simulink model "exampleModel_bus_axi_w_4ptavg"  (R2017b)
settings: Solver=VariableStepAuto  StartTime=0.0  StopTime=10e-5  RelTol=1e-3
PreLoadFcn:
  | setup
values from neighbouring files (symbols this model uses):
  axiClk = 156.25e6    (= 156250000)    [setup.m]    (also in setup_exampleModel_bus_axi_simulink.m; setup_exampleModel_bus_axi_simulink_lcls2.m; setup_lcls2_pcav.m; sysgen_signal.m)
  cav1p1_addr = 204    [setup_exampleModel_bus_axi_simulink.m]    (also in setup_exampleModel_bus_axi_simulink_lcls2.m; setup_lcls2_pcav.m; sysgen_signal.m)
  cav1p2_addr = cav1p1_addr * 2    (= 408)    [setup_exampleModel_bus_axi_simulink.m]    (also in setup_exampleModel_bus_axi_simulink_lcls2.m; setup_lcls2_pcav.m; sysgen_signal.m)
  cav2p1_addr = cav1p1_addr * 3    (= 612)    [setup_exampleModel_bus_axi_simulink.m]    (also in setup_exampleModel_bus_axi_simulink_lcls2.m; setup_lcls2_pcav.m; sysgen_signal.m)
  cav2p2_addr = cav1p1_addr * 4    (= 816)    [setup_exampleModel_bus_axi_simulink.m]    (also in setup_exampleModel_bus_axi_simulink_lcls2.m; setup_lcls2_pcav.m; sysgen_signal.m)
  Fadc = Fs/interleavedChannels    (= 29750000)    [setup.m]    (also in setup_exampleModel_bus_axi_simulink.m = 357000000; setup_exampleModel_bus_axi_simulink_lcls2.m = 351000000; setup_lcls2_pcav.m = 357000000; sysgen_signal.m = 357000000)
  fir_lpf = fir1(15, w_lpf)    [setup_exampleModel_bus_axi_simulink.m]    (also in setup_exampleModel_bus_axi_simulink_lcls2.m; setup_lcls2_pcav.m)
  Fproc = 204e6    (= 204000000)    [setup_exampleModel_bus_axi_simulink.m]    (also in setup_exampleModel_bus_axi_simulink_lcls2.m = 200571400; setup_lcls2_pcav.m; sysgen_signal.m)
  Fsig = Fproc/12    (= 17000000)    [setup_exampleModel_bus_axi_simulink.m]    (also in setup_exampleModel_bus_axi_simulink_lcls2.m = 16714283.3333; setup_lcls2_pcav.m)
  Tadc = 1/fadc    (= 2.80112044818e-09)    [cavity_signal.m]    (also in setup_exampleModel_bus_axi_simulink.m; setup_exampleModel_bus_axi_simulink_lcls2.m = 2.849002849e-09; setup_lcls2_pcav.m; setup_pcav_simulink.m)
undefined symbols (not defined in the file or in its folder): AXI4, Lite
libraries: xbsIndex_r4 x2870, llrf_lib x10, simulink x3
(part 4 of 15)

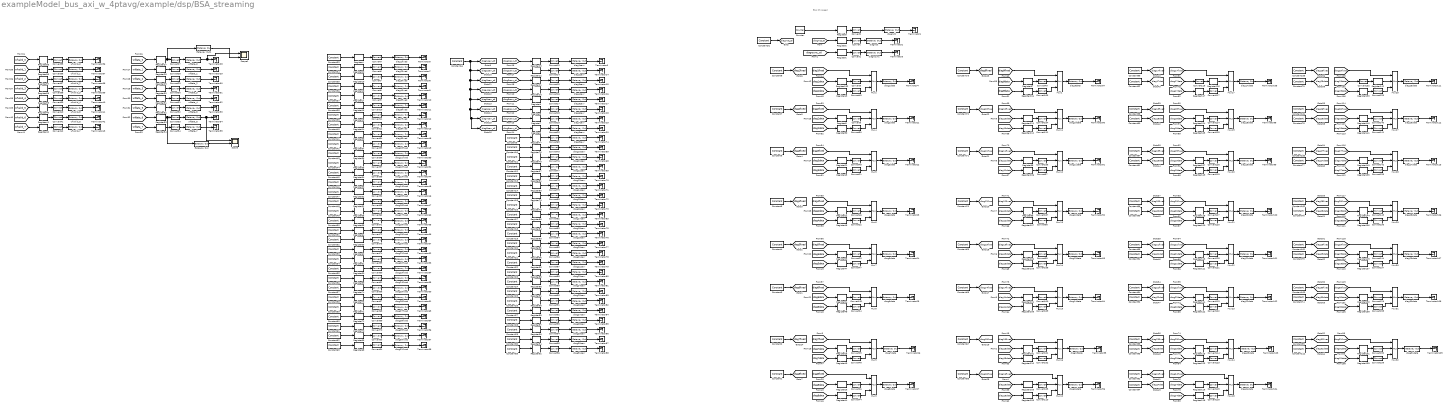
== system exampleModel_bus_axi_w_4ptavg/example/dsp/BSA_streaming ==
  note: BSA Clk speed
  Constant{1..8,66..73,82..89,99..105} (31 alike) : xbsIndex_r4/Constant  const=0  gui_display_data_type=Boolean  arith_type=Boolean  n_bits=16  bin_pt=14  preci_type=Single  exp_width=8  frac_width=24  explicit_period=off  period=1  equ=P=C  opselect=C  inp2=PCIN>>17  opr=+  inp1=P  carry=CIN  dbl_ovrd=off  block_type=constant
  Constant{9..30,64..65} (24 alike) : xbsIndex_r4/Constant  const=0  gui_display_data_type=Fixed-point  arith_type=Unsigned  n_bits=3  bin_pt=0  preci_type=Single  exp_width=8  frac_width=24  explicit_period=on  period=1/(17e6)  equ=P=C  opselect=C  inp2=PCIN>>17  opr=+  inp1=P  carry=CIN  dbl_ovrd=off  block_type=constant
  Constant{32,74..81,90..94,112} (15 alike) : xbsIndex_r4/Constant  const=0  gui_display_data_type=Fixed-point  arith_type=Signed (2's comp)  n_bits=18  bin_pt=0  preci_type=Single  exp_width=8  frac_width=24  explicit_period=on  period=1/Fproc  equ=P=C  opselect=C  inp2=PCIN>>17  opr=+  inp1=P  carry=CIN  dbl_ovrd=off  block_type=constant
  Constant31 : xbsIndex_r4/Constant  const=0  gui_display_data_type=Boolean  arith_type=Boolean  n_bits=16  bin_pt=14  preci_type=Single  exp_width=8  frac_width=24  explicit_period=on  period=1/(17e6)  equ=P=C  opselect=C  inp2=PCIN>>17  opr=+  inp1=P  carry=CIN  dbl_ovrd=off  block_type=constant
  Constant{33..63} (31 alike) : xbsIndex_r4/Constant  const=0  gui_display_data_type=Fixed-point  arith_type=Unsigned  n_bits=1  bin_pt=0  preci_type=Single  exp_width=8  frac_width=24  explicit_period=on  period=1/(17e6)  equ=P=C  opselect=C  inp2=PCIN>>17  opr=+  inp1=P  carry=CIN  dbl_ovrd=off  block_type=constant
  Convert{,1,4,6..12,35..42,51..64,66..74} (41 alike) : xbsIndex_r4/Convert  gui_display_data_type=Boolean  arith_type=Boolean  n_bits=16  bin_pt=14  float_type=Single  exp_bits=8  fraction_bits=24  quantization=Truncate  overflow=Wrap  en=off  latency=1  pipeline=off  dbl_ovrd=off  block_type=convert
  Convert{3,25,46,49,100..101,107,131} (8 alike) : xbsIndex_r4/Convert  gui_display_data_type=Fixed-point  arith_type="Signed  (2's comp)"  n_bits=18  bin_pt=16  float_type=Single  exp_bits=8  fraction_bits=24  quantization=Truncate  overflow=Wrap  en=off  latency=1  pipeline=off  dbl_ovrd=off  block_type=convert
  Convert{22,24,29..32,34,43,48,98,102..103,109} (13 alike) : xbsIndex_r4/Convert  gui_display_data_type=Fixed-point  arith_type="Signed  (2's comp)"  n_bits=32  bin_pt=16  float_type=Single  exp_bits=8  fraction_bits=24  quantization=Truncate  overflow=Wrap  en=off  latency=1  pipeline=off  dbl_ovrd=off  block_type=convert
  Convert{5,45,104,106} (4 alike) : xbsIndex_r4/Convert  gui_display_data_type=Fixed-point  arith_type="Signed  (2's comp)"  n_bits=18  bin_pt=15  float_type=Single  exp_bits=8  fraction_bits=24  quantization=Truncate  overflow=Wrap  en=off  latency=1  pipeline=off  dbl_ovrd=off  block_type=convert
  Convert{23,26,99,105,113..116,124,126..130,132,140,142..144} (19 alike) : xbsIndex_r4/Convert  gui_display_data_type=Fixed-point  arith_type="Signed  (2's comp)"  n_bits=18  bin_pt=0  float_type=Single  exp_bits=8  fraction_bits=24  quantization=Truncate  overflow=Wrap  en=off  latency=1  pipeline=off  dbl_ovrd=off  block_type=convert
  Convert{33,44,47,108,110,117..123,125,133,135..139,141} (20 alike) : xbsIndex_r4/Convert  gui_display_data_type=Fixed-point  arith_type="Signed  (2's comp)"  n_bits=32  bin_pt=0  float_type=Single  exp_bits=8  fraction_bits=24  quantization=Truncate  overflow=Wrap  en=off  latency=1  pipeline=off  dbl_ovrd=off  block_type=convert
  Convert{21,50,97,111} (4 alike) : xbsIndex_r4/Convert  gui_display_data_type=Fixed-point  arith_type="Signed  (2's comp)"  n_bits=32  bin_pt=15  float_type=Single  exp_bits=8  fraction_bits=24  quantization=Truncate  overflow=Wrap  en=off  latency=1  pipeline=off  dbl_ovrd=off  block_type=convert
  Convert{13..20,65,75..96} (31 alike) : xbsIndex_r4/Convert  gui_display_data_type=Fixed-point  arith_type=Unsigned  n_bits=2  bin_pt=0  float_type=Single  exp_bits=8  fraction_bits=24  quantization=Truncate  overflow=Wrap  en=off  latency=1  pipeline=off  dbl_ovrd=off  block_type=convert
  Convert2 : xbsIndex_r4/Convert  gui_display_data_type=Fixed-point  arith_type=Unsigned  n_bits=1  bin_pt=0  float_type=Single  exp_bits=8  fraction_bits=24  quantization=Truncate  overflow=Saturate  en=off  latency=1  pipeline=off  dbl_ovrd=off  block_type=convert
  Convert27 : xbsIndex_r4/Convert  gui_display_data_type=Fixed-point  arith_type="Signed  (2's comp)"  n_bits=32  bin_pt=24  float_type=Single  exp_bits=8  fraction_bits=24  quantization=Truncate  overflow=Wrap  en=off  latency=1  pipeline=off  dbl_ovrd=off  block_type=convert
  Convert28 : xbsIndex_r4/Convert  gui_display_data_type=Fixed-point  arith_type="Signed  (2's comp)"  n_bits=32  bin_pt=24  float_type=Single  exp_bits=8  fraction_bits=24  quantization=Truncate  overflow=Wrap  en=off  latency=1  pipeline=off  dbl_ovrd=off  block_type=convert
  Counter : xbsIndex_r4/Counter  cnt_type=Free Running  cnt_to=Inf  operation=Up  start_count=0  cnt_by_val=1  arith_type=Unsigned  n_bits=1  bin_pt=0  load_pin=off  rst=off  en=off  explicit_period=on  period=1/(Fproc)  use_behavioral_HDL=off  implementation=Fabric  dbl_ovrd=off  block_type=counter
  Gateway Out : xbsIndex_r4/Gateway Out  inherit_from_input=off  hdl_port=on  rows=1  columns=1  UseAsDAC=off  DACChannel='1'  interface=None  automatic_assignment=on  address_offset=hex2dec('00')  intf_name=''  intf_description=''  timing_constraint=None  locs_specified=off  LOCs={}  io_standard={}  block_type=gatewayout
  Gateway Out1 : xbsIndex_r4/Gateway Out  inherit_from_input=off  hdl_port=on  rows=1  columns=1  UseAsDAC=off  DACChannel='1'  interface=None  automatic_assignment=on  address_offset=hex2dec('00')  intf_name=''  intf_description=''  timing_constraint=None  locs_specified=off  LOCs={}  io_standard={}  block_type=gatewayout
  Mux{1..25,27..32} (31 alike) : xbsIndex_r4/Mux  inputs=2  en=off  latency=1  precision=Full  arith_type=Unsigned  n_bits=16  bin_pt=14  quantization=Truncate  overflow=Wrap  dbl_ovrd=off  block_type=mux
  Register{1..133,135..144} (143 alike) : xbsIndex_r4/Register  init=0  rst=off  en=off  dbl_ovrd=off  block_type=register
  Scope : Scope  NumInputPorts=2
  Scope1 : Scope  NumInputPorts=2
  Terminator{1..109,111..113} (112 alike) : Terminator
  diag10data : xbsIndex_r4/Gateway Out  inherit_from_input=off  hdl_port=on  rows=1  columns=1  UseAsDAC=off  DACChannel='1'  interface=None  automatic_assignment=on  address_offset=hex2dec('00')  intf_name=''  intf_description=''  timing_constraint=None  locs_specified=off  LOCs={}  io_standard={}  block_type=gatewayout
  diag10fixed : xbsIndex_r4/Gateway Out  inherit_from_input=off  hdl_port=on  rows=1  columns=1  UseAsDAC=off  DACChannel='1'  interface=None  automatic_assignment=on  address_offset=hex2dec('00')  intf_name=''  intf_description=''  timing_constraint=None  locs_specified=off  LOCs={}  io_standard={}  block_type=gatewayout
  diag10sevr : xbsIndex_r4/Gateway Out  inherit_from_input=off  hdl_port=on  rows=1  columns=1  UseAsDAC=off  DACChannel='1'  interface=None  automatic_assignment=on  address_offset=hex2dec('00')  intf_name=''  intf_description=''  timing_constraint=None  locs_specified=off  LOCs={}  io_standard={}  block_type=gatewayout
  diag11data : xbsIndex_r4/Gateway Out  inherit_from_input=off  hdl_port=on  rows=1  columns=1  UseAsDAC=off  DACChannel='1'  interface=None  automatic_assignment=on  address_offset=hex2dec('00')  intf_name=''  intf_description=''  timing_constraint=None  locs_specified=off  LOCs={}  io_standard={}  block_type=gatewayout
  diag11fixed : xbsIndex_r4/Gateway Out  inherit_from_input=off  hdl_port=on  rows=1  columns=1  UseAsDAC=off  DACChannel='1'  interface=None  automatic_assignment=on  address_offset=hex2dec('00')  intf_name=''  intf_description=''  timing_constraint=None  locs_specified=off  LOCs={}  io_standard={}  block_type=gatewayout
  diag11sevr : xbsIndex_r4/Gateway Out  inherit_from_input=off  hdl_port=on  rows=1  columns=1  UseAsDAC=off  DACChannel='1'  interface=None  automatic_assignment=on  address_offset=hex2dec('00')  intf_name=''  intf_description=''  timing_constraint=None  locs_specified=off  LOCs={}  io_standard={}  block_type=gatewayout
  diag12data : xbsIndex_r4/Gateway Out  inherit_from_input=off  hdl_port=on  rows=1  columns=1  UseAsDAC=off  DACChannel='1'  interface=None  automatic_assignment=on  address_offset=hex2dec('00')  intf_name=''  intf_description=''  timing_constraint=None  locs_specified=off  LOCs={}  io_standard={}  block_type=gatewayout
  diag12fixed : xbsIndex_r4/Gateway Out  inherit_from_input=off  hdl_port=on  rows=1  columns=1  UseAsDAC=off  DACChannel='1'  interface=None  automatic_assignment=on  address_offset=hex2dec('00')  intf_name=''  intf_description=''  timing_constraint=None  locs_specified=off  LOCs={}  io_standard={}  block_type=gatewayout
  diag12sevr : xbsIndex_r4/Gateway Out  inherit_from_input=off  hdl_port=on  rows=1  columns=1  UseAsDAC=off  DACChannel='1'  interface=None  automatic_assignment=on  address_offset=hex2dec('00')  intf_name=''  intf_description=''  timing_constraint=None  locs_specified=off  LOCs={}  io_standard={}  block_type=gatewayout
  diag13data : xbsIndex_r4/Gateway Out  inherit_from_input=off  hdl_port=on  rows=1  columns=1  UseAsDAC=off  DACChannel='1'  interface=None  automatic_assignment=on  address_offset=hex2dec('00')  intf_name=''  intf_description=''  timing_constraint=None  locs_specified=off  LOCs={}  io_standard={}  block_type=gatewayout
  diag13fixed : xbsIndex_r4/Gateway Out  inherit_from_input=off  hdl_port=on  rows=1  columns=1  UseAsDAC=off  DACChannel='1'  interface=None  automatic_assignment=on  address_offset=hex2dec('00')  intf_name=''  intf_description=''  timing_constraint=None  locs_specified=off  LOCs={}  io_standard={}  block_type=gatewayout
  diag13sevr : xbsIndex_r4/Gateway Out  inherit_from_input=off  hdl_port=on  rows=1  columns=1  UseAsDAC=off  DACChannel='1'  interface=None  automatic_assignment=on  address_offset=hex2dec('00')  intf_name=''  intf_description=''  timing_constraint=None  locs_specified=off  LOCs={}  io_standard={}  block_type=gatewayout
  diag14data : xbsIndex_r4/Gateway Out  inherit_from_input=off  hdl_port=on  rows=1  columns=1  UseAsDAC=off  DACChannel='1'  interface=None  automatic_assignment=on  address_offset=hex2dec('00')  intf_name=''  intf_description=''  timing_constraint=None  locs_specified=off  LOCs={}  io_standard={}  block_type=gatewayout
  diag14fixed : xbsIndex_r4/Gateway Out  inherit_from_input=off  hdl_port=on  rows=1  columns=1  UseAsDAC=off  DACChannel='1'  interface=None  automatic_assignment=on  address_offset=hex2dec('00')  intf_name=''  intf_description=''  timing_constraint=None  locs_specified=off  LOCs={}  io_standard={}  block_type=gatewayout
  diag14sevr : xbsIndex_r4/Gateway Out  inherit_from_input=off  hdl_port=on  rows=1  columns=1  UseAsDAC=off  DACChannel='1'  interface=None  automatic_assignment=on  address_offset=hex2dec('00')  intf_name=''  intf_description=''  timing_constraint=None  locs_specified=off  LOCs={}  io_standard={}  block_type=gatewayout
  diag15data : xbsIndex_r4/Gateway Out  inherit_from_input=off  hdl_port=on  rows=1  columns=1  UseAsDAC=off  DACChannel='1'  interface=None  automatic_assignment=on  address_offset=hex2dec('00')  intf_name=''  intf_description=''  timing_constraint=None  locs_specified=off  LOCs={}  io_standard={}  block_type=gatewayout
  diag15fixed : xbsIndex_r4/Gateway Out  inherit_from_input=off  hdl_port=on  rows=1  columns=1  UseAsDAC=off  DACChannel='1'  interface=None  automatic_assignment=on  address_offset=hex2dec('00')  intf_name=''  intf_description=''  timing_constraint=None  locs_specified=off  LOCs={}  io_standard={}  block_type=gatewayout
  diag15sevr : xbsIndex_r4/Gateway Out  inherit_from_input=off  hdl_port=on  rows=1  columns=1  UseAsDAC=off  DACChannel='1'  interface=None  automatic_assignment=on  address_offset=hex2dec('00')  intf_name=''  intf_description=''  timing_constraint=None  locs_specified=off  LOCs={}  io_standard={}  block_type=gatewayout
  diag16data : xbsIndex_r4/Gateway Out  inherit_from_input=off  hdl_port=on  rows=1  columns=1  UseAsDAC=off  DACChannel='1'  interface=None  automatic_assignment=on  address_offset=hex2dec('00')  intf_name=''  intf_description=''  timing_constraint=None  locs_specified=off  LOCs={}  io_standard={}  block_type=gatewayout
  diag16fixed : xbsIndex_r4/Gateway Out  inherit_from_input=off  hdl_port=on  rows=1  columns=1  UseAsDAC=off  DACChannel='1'  interface=None  automatic_assignment=on  address_offset=hex2dec('00')  intf_name=''  intf_description=''  timing_constraint=None  locs_specified=off  LOCs={}  io_standard={}  block_type=gatewayout
  diag16sevr : xbsIndex_r4/Gateway Out  inherit_from_input=off  hdl_port=on  rows=1  columns=1  UseAsDAC=off  DACChannel='1'  interface=None  automatic_assignment=on  address_offset=hex2dec('00')  intf_name=''  intf_description=''  timing_constraint=None  locs_specified=off  LOCs={}  io_standard={}  block_type=gatewayout
  diag17data : xbsIndex_r4/Gateway Out  inherit_from_input=off  hdl_port=on  rows=1  columns=1  UseAsDAC=off  DACChannel='1'  interface=None  automatic_assignment=on  address_offset=hex2dec('00')  intf_name=''  intf_description=''  timing_constraint=None  locs_specified=off  LOCs={}  io_standard={}  block_type=gatewayout
  diag17fixed : xbsIndex_r4/Gateway Out  inherit_from_input=off  hdl_port=on  rows=1  columns=1  UseAsDAC=off  DACChannel='1'  interface=None  automatic_assignment=on  address_offset=hex2dec('00')  intf_name=''  intf_description=''  timing_constraint=None  locs_specified=off  LOCs={}  io_standard={}  block_type=gatewayout
  diag17sevr : xbsIndex_r4/Gateway Out  inherit_from_input=off  hdl_port=on  rows=1  columns=1  UseAsDAC=off  DACChannel='1'  interface=None  automatic_assignment=on  address_offset=hex2dec('00')  intf_name=''  intf_description=''  timing_constraint=None  locs_specified=off  LOCs={}  io_standard={}  block_type=gatewayout
  diag18data : xbsIndex_r4/Gateway Out  inherit_from_input=off  hdl_port=on  rows=1  columns=1  UseAsDAC=off  DACChannel='1'  interface=None  automatic_assignment=on  address_offset=hex2dec('00')  intf_name=''  intf_description=''  timing_constraint=None  locs_specified=off  LOCs={}  io_standard={}  block_type=gatewayout
  diag18fixed : xbsIndex_r4/Gateway Out  inherit_from_input=off  hdl_port=on  rows=1  columns=1  UseAsDAC=off  DACChannel='1'  interface=None  automatic_assignment=on  address_offset=hex2dec('00')  intf_name=''  intf_description=''  timing_constraint=None  locs_specified=off  LOCs={}  io_standard={}  block_type=gatewayout
  diag18sevr : xbsIndex_r4/Gateway Out  inherit_from_input=off  hdl_port=on  rows=1  columns=1  UseAsDAC=off  DACChannel='1'  interface=None  automatic_assignment=on  address_offset=hex2dec('00')  intf_name=''  intf_description=''  timing_constraint=None  locs_specified=off  LOCs={}  io_standard={}  block_type=gatewayout
  diag19data : xbsIndex_r4/Gateway Out  inherit_from_input=off  hdl_port=on  rows=1  columns=1  UseAsDAC=off  DACChannel='1'  interface=None  automatic_assignment=on  address_offset=hex2dec('00')  intf_name=''  intf_description=''  timing_constraint=None  locs_specified=off  LOCs={}  io_standard={}  block_type=gatewayout
  diag19fixed : xbsIndex_r4/Gateway Out  inherit_from_input=off  hdl_port=on  rows=1  columns=1  UseAsDAC=off  DACChannel='1'  interface=None  automatic_assignment=on  address_offset=hex2dec('00')  intf_name=''  intf_description=''  timing_constraint=None  locs_specified=off  LOCs={}  io_standard={}  block_type=gatewayout
  diag19sevr : xbsIndex_r4/Gateway Out  inherit_from_input=off  hdl_port=on  rows=1  columns=1  UseAsDAC=off  DACChannel='1'  interface=None  automatic_assignment=on  address_offset=hex2dec('00')  intf_name=''  intf_description=''  timing_constraint=None  locs_specified=off  LOCs={}  io_standard={}  block_type=gatewayout
  diag1data : xbsIndex_r4/Gateway Out  inherit_from_input=off  hdl_port=on  rows=1  columns=1  UseAsDAC=off  DACChannel='1'  interface=None  automatic_assignment=on  address_offset=hex2dec('00')  intf_name=''  intf_description=''  timing_constraint=None  locs_specified=off  LOCs={}  io_standard={}  block_type=gatewayout
  diag1fixed : xbsIndex_r4/Gateway Out  inherit_from_input=off  hdl_port=on  rows=1  columns=1  UseAsDAC=off  DACChannel='1'  interface=None  automatic_assignment=on  address_offset=hex2dec('00')  intf_name=''  intf_description=''  timing_constraint=None  locs_specified=off  LOCs={}  io_standard={}  block_type=gatewayout
  diag1sevr : xbsIndex_r4/Gateway Out  inherit_from_input=off  hdl_port=on  rows=1  columns=1  UseAsDAC=off  DACChannel='1'  interface=None  automatic_assignment=on  address_offset=hex2dec('00')  intf_name=''  intf_description=''  timing_constraint=None  locs_specified=off  LOCs={}  io_standard={}  block_type=gatewayout
  diag20data : xbsIndex_r4/Gateway Out  inherit_from_input=off  hdl_port=on  rows=1  columns=1  UseAsDAC=off  DACChannel='1'  interface=None  automatic_assignment=on  address_offset=hex2dec('00')  intf_name=''  intf_description=''  timing_constraint=None  locs_specified=off  LOCs={}  io_standard={}  block_type=gatewayout
  diag20fixed : xbsIndex_r4/Gateway Out  inherit_from_input=off  hdl_port=on  rows=1  columns=1  UseAsDAC=off  DACChannel='1'  interface=None  automatic_assignment=on  address_offset=hex2dec('00')  intf_name=''  intf_description=''  timing_constraint=None  locs_specified=off  LOCs={}  io_standard={}  block_type=gatewayout
  diag20sevr : xbsIndex_r4/Gateway Out  inherit_from_input=off  hdl_port=on  rows=1  columns=1  UseAsDAC=off  DACChannel='1'  interface=None  automatic_assignment=on  address_offset=hex2dec('00')  intf_name=''  intf_description=''  timing_constraint=None  locs_specified=off  LOCs={}  io_standard={}  block_type=gatewayout
  diag21data : xbsIndex_r4/Gateway Out  inherit_from_input=off  hdl_port=on  rows=1  columns=1  UseAsDAC=off  DACChannel='1'  interface=None  automatic_assignment=on  address_offset=hex2dec('00')  intf_name=''  intf_description=''  timing_constraint=None  locs_specified=off  LOCs={}  io_standard={}  block_type=gatewayout
  diag21fixed : xbsIndex_r4/Gateway Out  inherit_from_input=off  hdl_port=on  rows=1  columns=1  UseAsDAC=off  DACChannel='1'  interface=None  automatic_assignment=on  address_offset=hex2dec('00')  intf_name=''  intf_description=''  timing_constraint=None  locs_specified=off  LOCs={}  io_standard={}  block_type=gatewayout
  diag21sevr : xbsIndex_r4/Gateway Out  inherit_from_input=off  hdl_port=on  rows=1  columns=1  UseAsDAC=off  DACChannel='1'  interface=None  automatic_assignment=on  address_offset=hex2dec('00')  intf_name=''  intf_description=''  timing_constraint=None  locs_specified=off  LOCs={}  io_standard={}  block_type=gatewayout
  diag22data : xbsIndex_r4/Gateway Out  inherit_from_input=off  hdl_port=on  rows=1  columns=1  UseAsDAC=off  DACChannel='1'  interface=None  automatic_assignment=on  address_offset=hex2dec('00')  intf_name=''  intf_description=''  timing_constraint=None  locs_specified=off  LOCs={}  io_standard={}  block_type=gatewayout
  diag22fixed : xbsIndex_r4/Gateway Out  inherit_from_input=off  hdl_port=on  rows=1  columns=1  UseAsDAC=off  DACChannel='1'  interface=None  automatic_assignment=on  address_offset=hex2dec('00')  intf_name=''  intf_description=''  timing_constraint=None  locs_specified=off  LOCs={}  io_standard={}  block_type=gatewayout
  diag22sevr : xbsIndex_r4/Gateway Out  inherit_from_input=off  hdl_port=on  rows=1  columns=1  UseAsDAC=off  DACChannel='1'  interface=None  automatic_assignment=on  address_offset=hex2dec('00')  intf_name=''  intf_description=''  timing_constraint=None  locs_specified=off  LOCs={}  io_standard={}  block_type=gatewayout
  diag23data : xbsIndex_r4/Gateway Out  inherit_from_input=off  hdl_port=on  rows=1  columns=1  UseAsDAC=off  DACChannel='1'  interface=None  automatic_assignment=on  address_offset=hex2dec('00')  intf_name=''  intf_description=''  timing_constraint=None  locs_specified=off  LOCs={}  io_standard={}  block_type=gatewayout
  diag23fixed : xbsIndex_r4/Gateway Out  inherit_from_input=off  hdl_port=on  rows=1  columns=1  UseAsDAC=off  DACChannel='1'  interface=None  automatic_assignment=on  address_offset=hex2dec('00')  intf_name=''  intf_description=''  timing_constraint=None  locs_specified=off  LOCs={}  io_standard={}  block_type=gatewayout
  diag23sevr : xbsIndex_r4/Gateway Out  inherit_from_input=off  hdl_port=on  rows=1  columns=1  UseAsDAC=off  DACChannel='1'  interface=None  automatic_assignment=on  address_offset=hex2dec('00')  intf_name=''  intf_description=''  timing_constraint=None  locs_specified=off  LOCs={}  io_standard={}  block_type=gatewayout
  diag24data : xbsIndex_r4/Gateway Out  inherit_from_input=off  hdl_port=on  rows=1  columns=1  UseAsDAC=off  DACChannel='1'  interface=None  automatic_assignment=on  address_offset=hex2dec('00')  intf_name=''  intf_description=''  timing_constraint=None  locs_specified=off  LOCs={}  io_standard={}  block_type=gatewayout
  diag24fixed : xbsIndex_r4/Gateway Out  inherit_from_input=off  hdl_port=on  rows=1  columns=1  UseAsDAC=off  DACChannel='1'  interface=None  automatic_assignment=on  address_offset=hex2dec('00')  intf_name=''  intf_description=''  timing_constraint=None  locs_specified=off  LOCs={}  io_standard={}  block_type=gatewayout
  diag24sevr : xbsIndex_r4/Gateway Out  inherit_from_input=off  hdl_port=on  rows=1  columns=1  UseAsDAC=off  DACChannel='1'  interface=None  automatic_assignment=on  address_offset=hex2dec('00')  intf_name=''  intf_description=''  timing_constraint=None  locs_specified=off  LOCs={}  io_standard={}  block_type=gatewayout
  diag25data : xbsIndex_r4/Gateway Out  inherit_from_input=off  hdl_port=on  rows=1  columns=1  UseAsDAC=off  DACChannel='1'  interface=None  automatic_assignment=on  address_offset=hex2dec('00')  intf_name=''  intf_description=''  timing_constraint=None  locs_specified=off  LOCs={}  io_standard={}  block_type=gatewayout
  diag25fixed : xbsIndex_r4/Gateway Out  inherit_from_input=off  hdl_port=on  rows=1  columns=1  UseAsDAC=off  DACChannel='1'  interface=None  automatic_assignment=on  address_offset=hex2dec('00')  intf_name=''  intf_description=''  timing_constraint=None  locs_specified=off  LOCs={}  io_standard={}  block_type=gatewayout
  diag25sevr : xbsIndex_r4/Gateway Out  inherit_from_input=off  hdl_port=on  rows=1  columns=1  UseAsDAC=off  DACChannel='1'  interface=None  automatic_assignment=on  address_offset=hex2dec('00')  intf_name=''  intf_description=''  timing_constraint=None  locs_specified=off  LOCs={}  io_standard={}  block_type=gatewayout
  diag26data : xbsIndex_r4/Gateway Out  inherit_from_input=off  hdl_port=on  rows=1  columns=1  UseAsDAC=off  DACChannel='1'  interface=None  automatic_assignment=on  address_offset=hex2dec('00')  intf_name=''  intf_description=''  timing_constraint=None  locs_specified=off  LOCs={}  io_standard={}  block_type=gatewayout
  diag26fixed : xbsIndex_r4/Gateway Out  inherit_from_input=off  hdl_port=on  rows=1  columns=1  UseAsDAC=off  DACChannel='1'  interface=None  automatic_assignment=on  address_offset=hex2dec('00')  intf_name=''  intf_description=''  timing_constraint=None  locs_specified=off  LOCs={}  io_standard={}  block_type=gatewayout
  diag26sevr : xbsIndex_r4/Gateway Out  inherit_from_input=off  hdl_port=on  rows=1  columns=1  UseAsDAC=off  DACChannel='1'  interface=None  automatic_assignment=on  address_offset=hex2dec('00')  intf_name=''  intf_description=''  timing_constraint=None  locs_specified=off  LOCs={}  io_standard={}  block_type=gatewayout
  diag27data : xbsIndex_r4/Gateway Out  inherit_from_input=off  hdl_port=on  rows=1  columns=1  UseAsDAC=off  DACChannel='1'  interface=None  automatic_assignment=on  address_offset=hex2dec('00')  intf_name=''  intf_description=''  timing_constraint=None  locs_specified=off  LOCs={}  io_standard={}  block_type=gatewayout
  diag27fixed : xbsIndex_r4/Gateway Out  inherit_from_input=off  hdl_port=on  rows=1  columns=1  UseAsDAC=off  DACChannel='1'  interface=None  automatic_assignment=on  address_offset=hex2dec('00')  intf_name=''  intf_description=''  timing_constraint=None  locs_specified=off  LOCs={}  io_standard={}  block_type=gatewayout
  diag27sevr : xbsIndex_r4/Gateway Out  inherit_from_input=off  hdl_port=on  rows=1  columns=1  UseAsDAC=off  DACChannel='1'  interface=None  automatic_assignment=on  address_offset=hex2dec('00')  intf_name=''  intf_description=''  timing_constraint=None  locs_specified=off  LOCs={}  io_standard={}  block_type=gatewayout
  diag28data : xbsIndex_r4/Gateway Out  inherit_from_input=off  hdl_port=on  rows=1  columns=1  UseAsDAC=off  DACChannel='1'  interface=None  automatic_assignment=on  address_offset=hex2dec('00')  intf_name=''  intf_description=''  timing_constraint=None  locs_specified=off  LOCs={}  io_standard={}  block_type=gatewayout
  diag28fixed : xbsIndex_r4/Gateway Out  inherit_from_input=off  hdl_port=on  rows=1  columns=1  UseAsDAC=off  DACChannel='1'  interface=None  automatic_assignment=on  address_offset=hex2dec('00')  intf_name=''  intf_description=''  timing_constraint=None  locs_specified=off  LOCs={}  io_standard={}  block_type=gatewayout
  diag28sevr : xbsIndex_r4/Gateway Out  inherit_from_input=off  hdl_port=on  rows=1  columns=1  UseAsDAC=off  DACChannel='1'  interface=None  automatic_assignment=on  address_offset=hex2dec('00')  intf_name=''  intf_description=''  timing_constraint=None  locs_specified=off  LOCs={}  io_standard={}  block_type=gatewayout
  diag29data : xbsIndex_r4/Gateway Out  inherit_from_input=off  hdl_port=on  rows=1  columns=1  UseAsDAC=off  DACChannel='1'  interface=None  automatic_assignment=on  address_offset=hex2dec('00')  intf_name=''  intf_description=''  timing_constraint=None  locs_specified=off  LOCs={}  io_standard={}  block_type=gatewayout
  diag29fixed : xbsIndex_r4/Gateway Out  inherit_from_input=off  hdl_port=on  rows=1  columns=1  UseAsDAC=off  DACChannel='1'  interface=None  automatic_assignment=on  address_offset=hex2dec('00')  intf_name=''  intf_description=''  timing_constraint=None  locs_specified=off  LOCs={}  io_standard={}  block_type=gatewayout
  diag29sevr : xbsIndex_r4/Gateway Out  inherit_from_input=off  hdl_port=on  rows=1  columns=1  UseAsDAC=off  DACChannel='1'  interface=None  automatic_assignment=on  address_offset=hex2dec('00')  intf_name=''  intf_description=''  timing_constraint=None  locs_specified=off  LOCs={}  io_standard={}  block_type=gatewayout
  diag2data : xbsIndex_r4/Gateway Out  inherit_from_input=off  hdl_port=on  rows=1  columns=1  UseAsDAC=off  DACChannel='1'  interface=None  automatic_assignment=on  address_offset=hex2dec('00')  intf_name=''  intf_description=''  timing_constraint=None  locs_specified=off  LOCs={}  io_standard={}  block_type=gatewayout
  diag2fixed : xbsIndex_r4/Gateway Out  inherit_from_input=off  hdl_port=on  rows=1  columns=1  UseAsDAC=off  DACChannel='1'  interface=None  automatic_assignment=on  address_offset=hex2dec('00')  intf_name=''  intf_description=''  timing_constraint=None  locs_specified=off  LOCs={}  io_standard={}  block_type=gatewayout
  diag2sevr : xbsIndex_r4/Gateway Out  inherit_from_input=off  hdl_port=on  rows=1  columns=1  UseAsDAC=off  DACChannel='1'  interface=None  automatic_assignment=on  address_offset=hex2dec('00')  intf_name=''  intf_description=''  timing_constraint=None  locs_specified=off  LOCs={}  io_standard={}  block_type=gatewayout
  diag30data : xbsIndex_r4/Gateway Out  inherit_from_input=off  hdl_port=on  rows=1  columns=1  UseAsDAC=off  DACChannel='1'  interface=None  automatic_assignment=on  address_offset=hex2dec('00')  intf_name=''  intf_description=''  timing_constraint=None  locs_specified=off  LOCs={}  io_standard={}  block_type=gatewayout
  diag30fixed : xbsIndex_r4/Gateway Out  inherit_from_input=off  hdl_port=on  rows=1  columns=1  UseAsDAC=off  DACChannel='1'  interface=None  automatic_assignment=on  address_offset=hex2dec('00')  intf_name=''  intf_description=''  timing_constraint=None  locs_specified=off  LOCs={}  io_standard={}  block_type=gatewayout
  diag30sevr : xbsIndex_r4/Gateway Out  inherit_from_input=off  hdl_port=on  rows=1  columns=1  UseAsDAC=off  DACChannel='1'  interface=None  automatic_assignment=on  address_offset=hex2dec('00')  intf_name=''  intf_description=''  timing_constraint=None  locs_specified=off  LOCs={}  io_standard={}  block_type=gatewayout
  diag31data : xbsIndex_r4/Gateway Out  inherit_from_input=off  hdl_port=on  rows=1  columns=1  UseAsDAC=off  DACChannel='1'  interface=None  automatic_assignment=on  address_offset=hex2dec('00')  intf_name=''  intf_description=''  timing_constraint=None  locs_specified=off  LOCs={}  io_standard={}  block_type=gatewayout
  diag31fixed : xbsIndex_r4/Gateway Out  inherit_from_input=off  hdl_port=on  rows=1  columns=1  UseAsDAC=off  DACChannel='1'  interface=None  automatic_assignment=on  address_offset=hex2dec('00')  intf_name=''  intf_description=''  timing_constraint=None  locs_specified=off  LOCs={}  io_standard={}  block_type=gatewayout
  diag31sevr : xbsIndex_r4/Gateway Out  inherit_from_input=off  hdl_port=on  rows=1  columns=1  UseAsDAC=off  DACChannel='1'  interface=None  automatic_assignment=on  address_offset=hex2dec('00')  intf_name=''  intf_description=''  timing_constraint=None  locs_specified=off  LOCs={}  io_standard={}  block_type=gatewayout
  diag3data : xbsIndex_r4/Gateway Out  inherit_from_input=off  hdl_port=on  rows=1  columns=1  UseAsDAC=off  DACChannel='1'  interface=None  automatic_assignment=on  address_offset=hex2dec('00')  intf_name=''  intf_description=''  timing_constraint=None  locs_specified=off  LOCs={}  io_standard={}  block_type=gatewayout
  diag3fixed : xbsIndex_r4/Gateway Out  inherit_from_input=off  hdl_port=on  rows=1  columns=1  UseAsDAC=off  DACChannel='1'  interface=None  automatic_assignment=on  address_offset=hex2dec('00')  intf_name=''  intf_description=''  timing_constraint=None  locs_specified=off  LOCs={}  io_standard={}  block_type=gatewayout
  diag3sevr : xbsIndex_r4/Gateway Out  inherit_from_input=off  hdl_port=on  rows=1  columns=1  UseAsDAC=off  DACChannel='1'  interface=None  automatic_assignment=on  address_offset=hex2dec('00')  intf_name=''  intf_description=''  timing_constraint=None  locs_specified=off  LOCs={}  io_standard={}  block_type=gatewayout
  diag4data : xbsIndex_r4/Gateway Out  inherit_from_input=off  hdl_port=on  rows=1  columns=1  UseAsDAC=off  DACChannel='1'  interface=None  automatic_assignment=on  address_offset=hex2dec('00')  intf_name=''  intf_description=''  timing_constraint=None  locs_specified=off  LOCs={}  io_standard={}  block_type=gatewayout
  diag4fixed : xbsIndex_r4/Gateway Out  inherit_from_input=off  hdl_port=on  rows=1  columns=1  UseAsDAC=off  DACChannel='1'  interface=None  automatic_assignment=on  address_offset=hex2dec('00')  intf_name=''  intf_description=''  timing_constraint=None  locs_specified=off  LOCs={}  io_standard={}  block_type=gatewayout
  diag4sevr : xbsIndex_r4/Gateway Out  inherit_from_input=off  hdl_port=on  rows=1  columns=1  UseAsDAC=off  DACChannel='1'  interface=None  automatic_assignment=on  address_offset=hex2dec('00')  intf_name=''  intf_description=''  timing_constraint=None  locs_specified=off  LOCs={}  io_standard={}  block_type=gatewayout
  diag5data : xbsIndex_r4/Gateway Out  inherit_from_input=off  hdl_port=on  rows=1  columns=1  UseAsDAC=off  DACChannel='1'  interface=None  automatic_assignment=on  address_offset=hex2dec('00')  intf_name=''  intf_description=''  timing_constraint=None  locs_specified=off  LOCs={}  io_standard={}  block_type=gatewayout
  diag5fixed : xbsIndex_r4/Gateway Out  inherit_from_input=off  hdl_port=on  rows=1  columns=1  UseAsDAC=off  DACChannel='1'  interface=None  automatic_assignment=on  address_offset=hex2dec('00')  intf_name=''  intf_description=''  timing_constraint=None  locs_specified=off  LOCs={}  io_standard={}  block_type=gatewayout
  diag5sevr : xbsIndex_r4/Gateway Out  inherit_from_input=off  hdl_port=on  rows=1  columns=1  UseAsDAC=off  DACChannel='1'  interface=None  automatic_assignment=on  address_offset=hex2dec('00')  intf_name=''  intf_description=''  timing_constraint=None  locs_specified=off  LOCs={}  io_standard={}  block_type=gatewayout
  diag6data : xbsIndex_r4/Gateway Out  inherit_from_input=off  hdl_port=on  rows=1  columns=1  UseAsDAC=off  DACChannel='1'  interface=None  automatic_assignment=on  address_offset=hex2dec('00')  intf_name=''  intf_description=''  timing_constraint=None  locs_specified=off  LOCs={}  io_standard={}  block_type=gatewayout
  diag6fixed : xbsIndex_r4/Gateway Out  inherit_from_input=off  hdl_port=on  rows=1  columns=1  UseAsDAC=off  DACChannel='1'  interface=None  automatic_assignment=on  address_offset=hex2dec('00')  intf_name=''  intf_description=''  timing_constraint=None  locs_specified=off  LOCs={}  io_standard={}  block_type=gatewayout
  diag6sevr : xbsIndex_r4/Gateway Out  inherit_from_input=off  hdl_port=on  rows=1  columns=1  UseAsDAC=off  DACChannel='1'  interface=None  automatic_assignment=on  address_offset=hex2dec('00')  intf_name=''  intf_description=''  timing_constraint=None  locs_specified=off  LOCs={}  io_standard={}  block_type=gatewayout
  diag7data : xbsIndex_r4/Gateway Out  inherit_from_input=off  hdl_port=on  rows=1  columns=1  UseAsDAC=off  DACChannel='1'  interface=None  automatic_assignment=on  address_offset=hex2dec('00')  intf_name=''  intf_description=''  timing_constraint=None  locs_specified=off  LOCs={}  io_standard={}  block_type=gatewayout
  diag7fixed : xbsIndex_r4/Gateway Out  inherit_from_input=off  hdl_port=on  rows=1  columns=1  UseAsDAC=off  DACChannel='1'  interface=None  automatic_assignment=on  address_offset=hex2dec('00')  intf_name=''  intf_description=''  timing_constraint=None  locs_specified=off  LOCs={}  io_standard={}  block_type=gatewayout
  diag7sevr : xbsIndex_r4/Gateway Out  inherit_from_input=off  hdl_port=on  rows=1  columns=1  UseAsDAC=off  DACChannel='1'  interface=None  automatic_assignment=on  address_offset=hex2dec('00')  intf_name=''  intf_description=''  timing_constraint=None  locs_specified=off  LOCs={}  io_standard={}  block_type=gatewayout
  diag8data : xbsIndex_r4/Gateway Out  inherit_from_input=off  hdl_port=on  rows=1  columns=1  UseAsDAC=off  DACChannel='1'  interface=None  automatic_assignment=on  address_offset=hex2dec('00')  intf_name=''  intf_description=''  timing_constraint=None  locs_specified=off  LOCs={}  io_standard={}  block_type=gatewayout
  diag8fixed : xbsIndex_r4/Gateway Out  inherit_from_input=off  hdl_port=on  rows=1  columns=1  UseAsDAC=off  DACChannel='1'  interface=None  automatic_assignment=on  address_offset=hex2dec('00')  intf_name=''  intf_description=''  timing_constraint=None  locs_specified=off  LOCs={}  io_standard={}  block_type=gatewayout
  diag8sevr : xbsIndex_r4/Gateway Out  inherit_from_input=off  hdl_port=on  rows=1  columns=1  UseAsDAC=off  DACChannel='1'  interface=None  automatic_assignment=on  address_offset=hex2dec('00')  intf_name=''  intf_description=''  timing_constraint=None  locs_specified=off  LOCs={}  io_standard={}  block_type=gatewayout
  diag9data : xbsIndex_r4/Gateway Out  inherit_from_input=off  hdl_port=on  rows=1  columns=1  UseAsDAC=off  DACChannel='1'  interface=None  automatic_assignment=on  address_offset=hex2dec('00')  intf_name=''  intf_description=''  timing_constraint=None  locs_specified=off  LOCs={}  io_standard={}  block_type=gatewayout
  diag9fixed : xbsIndex_r4/Gateway Out  inherit_from_input=off  hdl_port=on  rows=1  columns=1  UseAsDAC=off  DACChannel='1'  interface=None  automatic_assignment=on  address_offset=hex2dec('00')  intf_name=''  intf_description=''  timing_constraint=None  locs_specified=off  LOCs={}  io_standard={}  block_type=gatewayout
  diag9sevr : xbsIndex_r4/Gateway Out  inherit_from_input=off  hdl_port=on  rows=1  columns=1  UseAsDAC=off  DACChannel='1'  interface=None  automatic_assignment=on  address_offset=hex2dec('00')  intf_name=''  intf_description=''  timing_constraint=None  locs_specified=off  LOCs={}  io_standard={}  block_type=gatewayout
  diagnclk : xbsIndex_r4/Gateway Out  inherit_from_input=off  hdl_port=on  rows=1  columns=1  UseAsDAC=off  DACChannel='1'  interface=None  automatic_assignment=on  address_offset=hex2dec('00')  intf_name=''  intf_description=''  timing_constraint=None  locs_specified=off  LOCs={}  io_standard={}  block_type=gatewayout
  diagnrst : xbsIndex_r4/Gateway Out  inherit_from_input=off  hdl_port=on  rows=1  columns=1  UseAsDAC=off  DACChannel='1'  interface=None  automatic_assignment=on  address_offset=hex2dec('00')  intf_name=''  intf_description=''  timing_constraint=None  locs_specified=off  LOCs={}  io_standard={}  block_type=gatewayout
  diagnsync : xbsIndex_r4/Gateway Out  inherit_from_input=off  hdl_port=on  rows=1  columns=1  UseAsDAC=off  DACChannel='1'  interface=None  automatic_assignment=on  address_offset=hex2dec('00')  intf_name=''  intf_description=''  timing_constraint=None  locs_specified=off  LOCs={}  io_standard={}  block_type=gatewayout
  wfdata_{0..7} (8 alike) : xbsIndex_r4/Gateway Out  inherit_from_input=off  hdl_port=on  rows=1  columns=1  UseAsDAC=off  DACChannel='1'  interface=None  automatic_assignment=on  address_offset=hex2dec('00')  intf_name=''  intf_description=''  timing_constraint=None  locs_specified=off  LOCs={}  io_standard={}  block_type=gatewayout
  wfvalid_{0..7} (8 alike) : xbsIndex_r4/Gateway Out  inherit_from_input=off  hdl_port=on  rows=1  columns=1  UseAsDAC=off  DACChannel='1'  interface=None  automatic_assignment=on  address_offset=hex2dec('00')  intf_name=''  intf_description=''  timing_constraint=None  locs_specified=off  LOCs={}  io_standard={}  block_type=gatewayout
  tag scope: diag10fixed=global, diag11fixed=global, diag12fixed=global, diag13fixed=global, diag14fixed=global, diag15fixed=global, diag16fixed=global, diag17data=global, diag17fixed=global, diag18data=global, diag18fixed=global, diag19data=global, diag19fixed=global, diag1fixed=global, diag1sevr_ctl=global, diag20data=global, diag20fixed=global, diag21data=global, diag21fixed=global, diag22data=global, diag22fixed=global, diag23data=global, diag23fixed=global, diag24data=global, diag24fixed=global, diag25data=global, diag25fixed=global, diag26data=global, diag26fixed=global, diag27data=global, diag27fixed=global, diag28data=global, diag28fixed=global, diag29data=global, diag29fixed=global, diag2fixed=global, diag2sevr_ctl=global, diag30data=global, diag30fixed=global, diag31data=global, diag31fixed=global, diag3fixed=global, diag3sevr_ctl=global, diag4fixed=global, diag4sevr_ctl=global, diag5fixed=global, diag5sevr_ctl=global, diag6fixed=global, diag6sevr_ctl=global, diag7fixed=global, diag7sevr_ctl=global, diag8fixed=global, diag8sevr_ctl=global, diag9fixed=global, diagnrst_ctl=global
  wires:
  Register38/1 -> Convert38/1
  Register30/1 -> Convert30/1
  Convert42/1 -> wfvalid_7/1
  [wfvalid_2] -> Register37/1
  [wfvalid_1] -> Register36/1
  Convert40/1 -> wfvalid_5/1
  Convert39/1 -> wfvalid_4/1
  Register29/1 -> Convert29/1
  [wfdata_3] -> Register30/1
  wfvalid_4/1 -> Terminator40/1
  wfvalid_0/1 -> Terminator36/1
  [wfvalid_4] -> Register39/1
  [wfvalid_3] -> Register38/1
  Register41/1 -> Convert41/1
  wfvalid_3/1 -> Terminator39/1
  Convert27/1 -> wfdata_0/1
  Register37/1 -> Convert37/1
  wfvalid_6/1 -> Terminator42/1
  wfdata_3/1 -> Terminator31/1
  [wfdata_7] -> Register34/1
  Convert32/1 -> wfdata_5/1
  Convert33/1 -> wfdata_6/1
  [wfvalid_5] -> Register40/1
  [wfdata_1] -> Register28/1
  Register39/1 -> Convert39/1
  Register31/1 -> Convert31/1
  Convert34/1 -> wfdata_7/1
  wfvalid_1/1 -> Terminator37/1
  Register42/1 -> Convert42/1
  [wfvalid_0] -> Register35/1
  [wfvalid_7] -> Register42/1
  Convert38/1 -> wfvalid_3/1
  Register40/1 -> Convert40/1
  wfdata_0/1 -> Scope1/1, Terminator28/1
  wfdata_7/1 -> Terminator35/1
  Register32/1 -> Convert32/1
  [wfdata_4] -> Register31/1
  Register34/1 -> Convert34/1
  Convert37/1 -> wfvalid_2/1
  wfdata_5/1 -> Terminator33/1
  Convert41/1 -> wfvalid_6/1
  Convert28/1 -> wfdata_1/1
  [wfdata_6] -> Register33/1
  Convert31/1 -> wfdata_4/1
  Convert30/1 -> wfdata_3/1
  Convert36/1 -> wfvalid_1/1
  diag3sevr/1 -> Terminator15/1
  wfvalid_2/1 -> Terminator38/1
  wfdata_4/1 -> Terminator32/1
  [wfvalid_6] -> Register41/1
  diag6sevr/1 -> Terminator18/1
  diag5fixed/1 -> Terminator10/1
  Convert35/1 -> wfvalid_0/1
  diag5sevr/1 -> Terminator17/1
  diag4sevr/1 -> Terminator16/1
  wfdata_2/1 -> Terminator30/1
  diag7sevr/1 -> Terminator19/1
  [wfdata_2] -> Register29/1
  Register33/1 -> Gateway Out/1, Convert33/1
  diag2sevr/1 -> Terminator14/1
  Register36/1 -> Convert36/1
  wfdata_1/1 -> Terminator29/1
  diag6fixed/1 -> Terminator11/1
  Register28/1 -> Convert28/1
  diag8sevr/1 -> Terminator20/1
  diag4fixed/1 -> Terminator9/1
  wfvalid_7/1 -> Terminator43/1
  [wfdata_5] -> Register32/1
  Convert29/1 -> wfdata_2/1
  Register27/1 -> Gateway Out1/1, Convert27/1
  diag7fixed/1 -> Terminator12/1
  diag8fixed/1 -> Terminator13/1
  [wfdata_0] -> Register27/1
  wfvalid_5/1 -> Terminator41/1
  Register35/1 -> Convert35/1
  diag2fixed/1 -> Terminator7/1
  diag3fixed/1 -> Terminator8/1
  wfdata_6/1 -> Scope/1, Terminator34/1
  Convert4/1 -> diag1fixed/1
  Constant33/1 -> Register4/1
  diag1fixed/1 -> Terminator5/1
  diag1sevr/1 -> Terminator6/1
  Constant34/1 -> Register20/1
  Constant35/1 -> Register19/1
  Constant36/1 -> Register18/1
  Constant37/1 -> Register17/1
  Constant38/1 -> Register16/1
  Constant39/1 -> Register15/1
  Constant40/1 -> Register14/1
  [diag1sevr_ctl] -> Register13/1
  [diag2sevr_ctl] -> Register12/1
  [diag3sevr_ctl] -> Register11/1
  [diag4sevr_ctl] -> Register10/1
  [diag5sevr_ctl] -> Register9/1
  [diag6sevr_ctl] -> Register8/1
  [diag7sevr_ctl] -> Register7/1
  [diag8sevr_ctl] -> Register6/1
  Convert6/1 -> diag2fixed/1
  Convert7/1 -> diag3fixed/1
  Convert8/1 -> diag4fixed/1
  Convert9/1 -> diag5fixed/1
  Convert10/1 -> diag6fixed/1
  Convert11/1 -> diag7fixed/1
  Convert12/1 -> diag8fixed/1
  Convert13/1 -> diag1sevr/1
  Convert14/1 -> diag2sevr/1
  Convert15/1 -> diag3sevr/1
  Convert16/1 -> diag4sevr/1
  Convert17/1 -> diag5sevr/1
  Convert18/1 -> diag6sevr/1
  Convert19/1 -> diag7sevr/1
  Convert20/1 -> diag8sevr/1
  Register4/1 -> Convert4/1
  Register6/1 -> Convert20/1
  Register7/1 -> Convert19/1
  Register8/1 -> Convert18/1
  Register9/1 -> Convert17/1
  Register10/1 -> Convert16/1
  Register11/1 -> Convert15/1
  Register12/1 -> Convert14/1
  Register13/1 -> Convert13/1
  Register14/1 -> Convert12/1
  Register15/1 -> Convert11/1
  Register16/1 -> Convert10/1
  Register17/1 -> Convert9/1
  Register18/1 -> Convert8/1
  Register19/1 -> Convert7/1
  Register20/1 -> Convert6/1
  Convert26/1 -> Mux3/2
  Convert2/1 -> diagnclk/1
  Convert45/1 -> Mux5/2
  Convert131/1 -> Mux8/2
  diag5data/1 -> Terminator24/1
  Register22/1 -> Convert46/1
  [diag1data] -> Register132/1
  Convert50/1 -> Mux4/3
  Register1/1 -> Convert1/1
  Convert24/1 -> Mux8/3
  [diag4fixed] -> Mux6/1
  Constant7/1 -> [diag2fixed]
  Mux7/1 -> diag5data/1
  Register45/1 -> Convert21/1
  Register25/1 -> Convert25/1
  [diagnsync_ctl] -> Register1/1
  Convert1/1 -> diagnsync/1
  Convert/1 -> diagnrst/1
  [diag2fixed] -> Mux4/1
  Constant8/1 -> [diag1fixed]
  [diag3fixed] -> Mux5/1
  diag1data/1 -> Terminator4/1
  [diag8data] -> Register26/1
  [diag3data] -> Register45/1
  Convert43/1 -> Mux2/3
  Register21/1 -> Convert45/1
  Register49/1 -> Convert48/1
  Convert47/1 -> Mux7/3
  diagnsync/1 -> Terminator3/1
  Mux4/1 -> diag2data/1
  [diag1fixed] -> Mux2/1
  Convert25/1 -> Mux9/2
  [diag7data] -> Register49/1
  Mux5/1 -> diag3data/1
  Constant6/1 -> [diag3fixed]
  diagnclk/1 -> Terminator1/1
  [diag5fixed] -> Mux7/1
  Convert5/1 -> Mux4/2
  Mux8/1 -> diag6data/1
  Convert46/1 -> Mux6/2
  Constant1/1 -> [diag8fixed]
  Constant5/1 -> [diag4fixed]
  [diag2data] -> Register5/1
  Mux6/1 -> diag4data/1
  Constant3/1 -> [diag6fixed]
  Mux3/1 -> diag8data/1
  Register5/1 -> Convert5/1
  Constant2/1 -> [diag7fixed]
  [diagnrst_ctl] -> Register2/1
  [diag4data] -> Register22/1
  Register26/1 -> Convert26/1
  [diag4data] -> Register46/1
  Register24/1 -> Convert131/1
  Mux9/1 -> diag7data/1
  Constant4/1 -> [diag5fixed]
  diag3data/1 -> Terminator22/1
  [diag5data] -> Register47/1
  [diag7fixed] -> Mux9/1
  Register2/1 -> Convert/1
  Register48/1 -> Convert24/1
  [diag6data] -> Register48/1
  [diag2data] -> Register50/1
  Register46/1 -> Convert22/1
  [diag6data] -> Register24/1
  Register23/1 -> Convert23/1
  diagnrst/1 -> Terminator2/1
  Convert23/1 -> Mux7/2
  [diag3data] -> Register21/1
  Register50/1 -> Convert50/1
  diag6data/1 -> Terminator25/1
  diag4data/1 -> Terminator23/1
  Mux2/1 -> diag1data/1
  [diag6fixed] -> Mux8/1
  Register47/1 -> Convert47/1
  Register43/1 -> Convert43/1
  diag8data/1 -> Terminator27/1
  [diag8data] -> Register44/1
  Convert21/1 -> Mux5/3
  Convert48/1 -> Mux9/3
  Convert44/1 -> Mux3/3
  [diag8fixed] -> Mux3/1
  [diag1data] -> Register43/1
  [diag5data] -> Register23/1
  diag2data/1 -> Terminator21/1
  [diag7data] -> Register25/1
  Convert22/1 -> Mux6/3
  diag7data/1 -> Terminator26/1
  Register3/1 -> Convert2/1
  Register44/1 -> Convert44/1
  Register57/1 -> Convert55/1
  Register56/1 -> Convert56/1
  Register55/1 -> Convert57/1
  Register54/1 -> Convert58/1
  Register53/1 -> Convert51/1
  Register52/1 -> Convert52/1
  Register51/1 -> Convert53/1
  Register58/1 -> Convert54/1
  Convert53/1 -> diag16fixed/1
  Convert52/1 -> diag15fixed/1
  Convert51/1 -> diag14fixed/1
  Convert58/1 -> diag13fixed/1
  Convert57/1 -> diag12fixed/1
  Convert56/1 -> diag11fixed/1
  Convert55/1 -> diag10fixed/1
  Constant48/1 -> Register51/1
  Constant47/1 -> Register52/1
  Constant46/1 -> Register53/1
  Constant45/1 -> Register54/1
  Constant44/1 -> Register55/1
  Constant43/1 -> Register56/1
  Constant42/1 -> Register57/1
  diag9fixed/1 -> Terminator48/1
  Constant41/1 -> Register58/1
  Convert54/1 -> diag9fixed/1
  diag11fixed/1 -> Terminator50/1
  diag10fixed/1 -> Terminator49/1
  diag16fixed/1 -> Terminator47/1
  diag15fixed/1 -> Terminator46/1
  diag12fixed/1 -> Terminator51/1
  diag14fixed/1 -> Terminator45/1
  diag13fixed/1 -> Terminator44/1
  diag29fixed/1 -> Terminator56/1
  diag30fixed/1 -> Terminator57/1
  diag28fixed/1 -> Terminator64/1
  diag31fixed/1 -> Terminator58/1
  diag26fixed/1 -> Terminator61/1
  diag27fixed/1 -> Terminator63/1
  Convert66/1 -> diag25fixed/1
  Constant57/1 -> Register74/1
  diag25fixed/1 -> Terminator60/1
  Constant58/1 -> Register73/1
  Constant59/1 -> Register72/1
  Constant60/1 -> Register71/1
  Constant61/1 -> Register70/1
  Constant62/1 -> Register69/1
  Constant63/1 -> Register68/1
  Convert67/1 -> diag26fixed/1
  Convert68/1 -> diag27fixed/1
  Convert69/1 -> diag28fixed/1
  Convert70/1 -> diag29fixed/1
  Convert63/1 -> diag30fixed/1
  Convert64/1 -> diag31fixed/1
  Register74/1 -> Convert66/1
  Register68/1 -> Convert64/1
  Register69/1 -> Convert63/1
  Register70/1 -> Convert70/1
  Register71/1 -> Convert69/1
  Register72/1 -> Convert68/1
  Register73/1 -> Convert67/1
  Register65/1 -> Convert71/1
  Register64/1 -> Convert72/1
  Register63/1 -> Convert73/1
  Register62/1 -> Convert74/1
  Register61/1 -> Convert59/1
  Register60/1 -> Convert60/1
  Register59/1 -> Convert61/1
  Register66/1 -> Convert62/1
  Convert61/1 -> diag24fixed/1
  Convert60/1 -> diag23fixed/1
  Convert59/1 -> diag22fixed/1
  Convert74/1 -> diag21fixed/1
  Convert73/1 -> diag20fixed/1
  Convert72/1 -> diag19fixed/1
  Convert71/1 -> diag18fixed/1
  Constant56/1 -> Register59/1
  Constant55/1 -> Register60/1
  Constant54/1 -> Register61/1
  Constant53/1 -> Register62/1
  Constant52/1 -> Register63/1
  Constant51/1 -> Register64/1
  Constant50/1 -> Register65/1
  diag17fixed/1 -> Terminator62/1
  Constant49/1 -> Register66/1
  Convert62/1 -> diag17fixed/1
  diag19fixed/1 -> Terminator66/1
  diag18fixed/1 -> Terminator65/1
  diag24fixed/1 -> Terminator55/1
  diag23fixed/1 -> Terminator54/1
  diag20fixed/1 -> Terminator67/1
  diag22fixed/1 -> Terminator53/1
  diag21fixed/1 -> Terminator52/1
  Register77/1 -> Convert65/1
  Register76/1 -> Convert75/1
  Register75/1 -> Convert76/1
  Register67/1 -> Convert77/1
  Register81/1 -> Convert78/1
  Register80/1 -> Convert79/1
  Register79/1 -> Convert80/1
  Register78/1 -> Convert81/1
  Convert81/1 -> diag16sevr/1
  Convert80/1 -> diag15sevr/1
  Convert79/1 -> diag14sevr/1
  Convert78/1 -> diag13sevr/1
  Convert77/1 -> diag12sevr/1
  Convert76/1 -> diag11sevr/1
  Convert75/1 -> diag10sevr/1
  Convert65/1 -> diag9sevr/1
  Constant16/1 -> Register78/1
  Constant15/1 -> Register79/1
  Constant14/1 -> Register80/1
  Constant13/1 -> Register81/1
  Constant12/1 -> Register67/1
  Constant11/1 -> Register75/1
  Constant10/1 -> Register76/1
  Constant9/1 -> Register77/1
  diag9sevr/1 -> Terminator74/1
  diag16sevr/1 -> Terminator73/1
  diag10sevr/1 -> Terminator59/1
  diag15sevr/1 -> Terminator72/1
  diag12sevr/1 -> Terminator69/1
  diag13sevr/1 -> Terminator70/1
  diag14sevr/1 -> Terminator71/1
  diag11sevr/1 -> Terminator68/1
  diag27sevr/1 -> Terminator84/1
  diag30sevr/1 -> Terminator87/1
  diag29sevr/1 -> Terminator86/1
  diag28sevr/1 -> Terminator85/1
  diag31sevr/1 -> Terminator88/1
  diag26sevr/1 -> Terminator82/1
  diag25sevr/1 -> Terminator89/1
  Constant25/1 -> Register91/1
  Constant26/1 -> Register90/1
  Constant27/1 -> Register89/1
  Constant28/1 -> Register87/1
  Constant29/1 -> Register95/1
  Constant30/1 -> Register94/1
  Constant65/1 -> Register92/1
  Convert90/1 -> diag25sevr/1
  Convert91/1 -> diag26sevr/1
  Convert92/1 -> diag27sevr/1
  Convert93/1 -> diag28sevr/1
  Convert94/1 -> diag29sevr/1
  Convert95/1 -> diag30sevr/1
  Convert96/1 -> diag31sevr/1
  Register92/1 -> Convert96/1
  Register94/1 -> Convert95/1
  Register95/1 -> Convert94/1
  Register87/1 -> Convert93/1
  Register89/1 -> Convert92/1
  Register90/1 -> Convert91/1
  Register91/1 -> Convert90/1
  Register85/1 -> Convert82/1
  Register84/1 -> Convert83/1
  Register83/1 -> Convert84/1
  Register82/1 -> Convert85/1
  Register96/1 -> Convert86/1
  Register93/1 -> Convert87/1
  Register88/1 -> Convert88/1
  Register86/1 -> Convert89/1
  Convert89/1 -> diag24sevr/1
  Convert88/1 -> diag23sevr/1
  Convert87/1 -> diag22sevr/1
  Convert86/1 -> diag21sevr/1
  Convert85/1 -> diag20sevr/1
  Convert84/1 -> diag19sevr/1
  Convert83/1 -> diag18sevr/1
  Convert82/1 -> diag17sevr/1
  Constant24/1 -> Register86/1
  Constant23/1 -> Register88/1
  Constant22/1 -> Register93/1
  Constant21/1 -> Register96/1
  Constant20/1 -> Register82/1
  Constant19/1 -> Register83/1
  Constant18/1 -> Register84/1
  Constant17/1 -> Register85/1
  diag17sevr/1 -> Terminator83/1
  diag24sevr/1 -> Terminator81/1
  diag18sevr/1 -> Terminator75/1
  diag23sevr/1 -> Terminator80/1
  diag20sevr/1 -> Terminator77/1
  diag21sevr/1 -> Terminator78/1
  diag22sevr/1 -> Terminator79/1
  diag19sevr/1 -> Terminator76/1
  Counter/1 -> Register3/1
  Constant31/1 -> [diagnrst_ctl]
  Constant64/1 -> [diag8sevr_ctl], [diag7sevr_ctl], [diag6sevr_ctl], [diag5sevr_ctl], [diag4sevr_ctl], [diag3sevr_ctl], [diag2sevr_ctl], [diag1sevr_ctl]
  [diag9data] -> Register97/1
  Register105/1 -> Convert110/1
  diag15data/1 -> Terminator95/1
  Convert98/1 -> Mux13/3
  [diag15data] -> Register102/1
  diag10data/1 -> Terminator90/1
  [diag13data] -> Register100/1
  [diag9data] -> Register104/1
  [diag16fixed] -> Mux10/1
  Convert110/1 -> Mux10/3
  Convert102/1 -> Mux16/3
  Convert97/1 -> Mux12/3
  [diag16data] -> Register105/1
  diag16data/1 -> Terminator96/1
  Register104/1 -> Convert103/1
  Register108/1 -> Convert108/1
  [diag14fixed] -> Mux15/1
  Mux1/1 -> diag9data/1
  diag12data/1 -> Terminator92/1
  diag14data/1 -> Terminator94/1
  Register112/1 -> Convert111/1
  [diag11data] -> Register98/1
  Convert99/1 -> Mux14/2
  Register100/1 -> Convert99/1
  [diag14data] -> Register101/1
  Register107/1 -> Convert98/1
  [diag10data] -> Register112/1
  [diag14data] -> Register109/1
  Register109/1 -> Convert109/1
  [diag15fixed] -> Mux16/1
  [diag13data] -> Register108/1
  diag11data/1 -> Terminator91/1
  Constant69/1 -> [diag13fixed]
  Mux16/1 -> diag15data/1
  Register101/1 -> Convert100/1
  [diag12data] -> Register107/1
  Register103/1 -> Convert105/1
  [diag12data] -> Register99/1
  Constant67/1 -> [diag15fixed]
  Register111/1 -> Convert104/1
  Mux10/1 -> diag16data/1
  Constant68/1 -> [diag14fixed]
  Mux13/1 -> diag12data/1
  [diag10data] -> Register111/1
  Constant70/1 -> [diag12fixed]
  Constant66/1 -> [diag16fixed]
  Convert107/1 -> Mux13/2
  Mux15/1 -> diag14data/1
  Convert104/1 -> Mux11/2
  [diag13fixed] -> Mux14/1
  Constant71/1 -> [diag11fixed]
  Mux12/1 -> diag11data/1
  [diag15data] -> Register110/1
  Convert101/1 -> Mux16/2
  [diag9fixed] -> Mux1/1
  Mux11/1 -> diag10data/1
  Convert108/1 -> Mux14/3
  Register110/1 -> Convert102/1
  Register98/1 -> Convert106/1
  Convert103/1 -> Mux1/3
  [diag11data] -> Register106/1
  [diag16data] -> Register103/1
  diag9data/1 -> Terminator97/1
  [diag11fixed] -> Mux12/1
  Constant73/1 -> [diag9fixed]
  [diag10fixed] -> Mux11/1
  Register102/1 -> Convert101/1
  Register106/1 -> Convert97/1
  Mux14/1 -> diag13data/1
  Constant72/1 -> [diag10fixed]
  [diag12fixed] -> Mux13/1
  Register97/1 -> Convert49/1
  Convert109/1 -> Mux15/3
  Convert111/1 -> Mux11/3
  Register99/1 -> Convert107/1
  diag13data/1 -> Terminator93/1
  Convert100/1 -> Mux15/2
  Convert106/1 -> Mux12/2
  Convert105/1 -> Mux10/2
  Convert115/1 -> Mux18/2
  Convert126/1 -> Mux20/2
  Convert113/1 -> Mux23/2
  diag21data/1 -> Terminator101/1
  Register128/1 -> Convert127/1
  [diag17data] -> Convert116/1
  Convert125/1 -> Mux19/3
  Convert122/1 -> Mux23/3
  Register126/1 -> Mux17/2
  [diag20fixed] -> Mux21/1
  Constant88/1 -> [diag18fixed]
  Mux22/1 -> diag21data/1
  Register119/1 -> Convert119/1
  Register115/1 -> Convert114/1
  [diag18fixed] -> Mux19/1
  Constant89/1 -> [diag17fixed]
  [diag19fixed] -> Mux20/1
  diag17data/1 -> Terminator105/1
  [diag24data] -> Register116/1
  [diag19data] -> Register119/1
  Convert117/1 -> Mux17/3
  Register127/1 -> Convert126/1
  Register123/1 -> Convert123/1
  Convert121/1 -> Mux22/3
  Mux19/1 -> diag18data/1
  [diag17fixed] -> Mux17/1
  Convert114/1 -> Mux24/2
  [diag23data] -> Register123/1
  Mux20/1 -> diag19data/1
  Constant87/1 -> [diag19fixed]
  [diag21fixed] -> Mux22/1
  Convert124/1 -> Mux19/2
  Mux23/1 -> diag22data/1
  Convert127/1 -> Mux21/2
  Constant82/1 -> [diag24fixed]
  Constant86/1 -> [diag20fixed]
  [diag18data] -> Register124/1
  Mux21/1 -> diag20data/1
  Constant84/1 -> [diag22fixed]
  Mux18/1 -> diag24data/1
  Register124/1 -> Convert124/1
  Constant83/1 -> [diag23fixed]
  [diag20data] -> Register128/1
  Register116/1 -> Convert115/1
  [diag20data] -> Register120/1
  Register114/1 -> Convert113/1
  Mux24/1 -> diag23data/1
  Constant85/1 -> [diag21fixed]
  diag19data/1 -> Terminator99/1
  [diag21data] -> Register121/1
  [diag23fixed] -> Mux24/1
  Register122/1 -> Convert122/1
  [diag22data] -> Register122/1
  [diag18data] -> Register125/1
  Register120/1 -> Convert120/1
  [diag22data] -> Register114/1
  Register113/1 -> Convert128/1
  Convert128/1 -> Mux22/2
  [diag19data] -> Register127/1
  Register125/1 -> Convert125/1
  diag22data/1 -> Terminator102/1
  diag20data/1 -> Terminator100/1
  Mux17/1 -> diag17data/1
  [diag22fixed] -> Mux23/1
  Register121/1 -> Convert121/1
  Register117/1 -> Convert117/1
  diag24data/1 -> Terminator104/1
  [diag24data] -> Register118/1
  Convert119/1 -> Mux20/3
  Convert123/1 -> Mux24/3
  Convert118/1 -> Mux18/3
  [diag24fixed] -> Mux18/1
  [diag17data] -> Register117/1
  [diag21data] -> Register113/1
  diag18data/1 -> Terminator98/1
  [diag23data] -> Register115/1
  Convert120/1 -> Mux21/3
  diag23data/1 -> Terminator103/1
  Register118/1 -> Convert118/1
  Convert116/1 -> Register126/1
  Convert132/1 -> Register142/1
  diag31data/1 -> Terminator109/1
  Convert136/1 -> Mux29/3
  [diag31data] -> Register131/1
  diag26data/1 -> Terminator112/1
  [diag29data] -> Register129/1
  [diag25data] -> Register133/1
  Convert139/1 -> Mux32/3
  Convert135/1 -> Mux28/3
  Register133/1 -> Convert133/1
  Register137/1 -> Convert137/1
  [diag30fixed] -> Mux31/1
  Mux25/1 -> diag25data/1
  diag28data/1 -> Terminator106/1
  diag30data/1 -> Terminator108/1
  Register141/1 -> Convert141/1
  [diag27data] -> Register143/1
  Convert144/1 -> Mux30/2
  Register129/1 -> Convert144/1
  [diag30data] -> Register130/1
  Register136/1 -> Convert136/1
  [diag26data] -> Register141/1
  [diag30data] -> Register138/1
  Register138/1 -> Convert138/1
  [diag31fixed] -> Mux32/1
  [diag29data] -> Register137/1
  diag27data/1 -> Terminator113/1
  Constant101/1 -> [diag29fixed]
  Mux32/1 -> diag31data/1
  Register130/1 -> Convert129/1
  [diag28data] -> Register136/1
  [diag28data] -> Register144/1
  Constant99/1 -> [diag31fixed]
  Register140/1 -> Convert140/1
  Constant100/1 -> [diag30fixed]
  Mux29/1 -> diag28data/1
  [diag26data] -> Register140/1
  Constant102/1 -> [diag28fixed]
  Convert143/1 -> Mux29/2
  Mux31/1 -> diag30data/1
  Convert140/1 -> Mux27/2
  [diag29fixed] -> Mux30/1
  Constant103/1 -> [diag27fixed]
  Mux28/1 -> diag27data/1
  [diag31data] -> Register139/1
  Convert130/1 -> Mux32/2
  [diag25fixed] -> Mux25/1
  Mux27/1 -> diag26data/1
  Convert137/1 -> Mux30/3
  Register139/1 -> Convert139/1
  Register143/1 -> Convert142/1
  Convert133/1 -> Mux25/3
  [diag27data] -> Register135/1
  diag25data/1 -> Terminator111/1
  [diag27fixed] -> Mux28/1
  Constant105/1 -> [diag25fixed]
  [diag26fixed] -> Mux27/1
  Register131/1 -> Convert130/1
  Register135/1 -> Convert135/1
  Mux30/1 -> diag29data/1
  Constant104/1 -> [diag26fixed]
  [diag28fixed] -> Mux29/1
  Register142/1 -> Mux25/2
  Convert138/1 -> Mux31/3
  Convert141/1 -> Mux27/3
  [diag25data] -> Convert132/1
  Register144/1 -> Convert143/1
  diag29data/1 -> Terminator107/1
  Convert129/1 -> Mux31/2
  Convert142/1 -> Mux28/2
  Constant79/1 -> [diag25data]
  Constant78/1 -> [diag26data]
  Constant77/1 -> [diag27data]
  Constant76/1 -> [diag28data]
  Constant75/1 -> [diag29data]
  Constant74/1 -> [diag30data]
  Constant112/1 -> [diag31data]
  Constant32/1 -> [diag17data]
  Constant80/1 -> [diag18data]
  Constant81/1 -> [diag19data]
  Constant90/1 -> [diag20data]
  Constant91/1 -> [diag21data]
  Constant92/1 -> [diag22data]
  Constant93/1 -> [diag23data]
  Constant94/1 -> [diag24data]
  Gateway Out/1 -> Scope/2
  Gateway Out1/1 -> Scope1/2
  Convert3/1 -> Mux2/2
  Register132/1 -> Convert3/1
  Convert49/1 -> Mux1/2
